simulink subsystem "EnergyElectroThermal"  (R2023b)
settings: Solver=VariableStepAuto  StartTime=0.0  StopTime=10.0  RelTol=1e-3
settings Model: Creator=jjha  LastModifiedBy=jjha

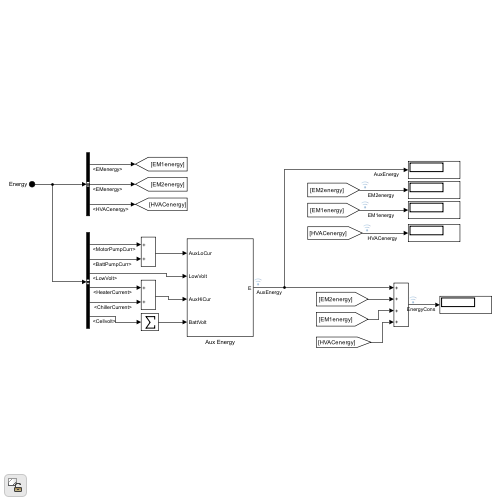
[thumbnail: Simulink's stored preview of the top-level diagram]
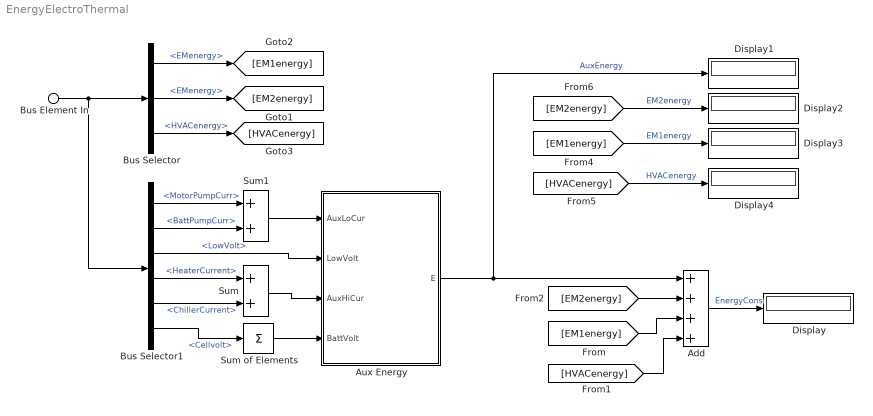
== system EnergyElectroThermal ==
  Bus Element In : Inport  PortName=Energy
  Add : Sum  Inputs=++++
  Aux Energy : Subsystem
  Bus Selector : BusSelector  OutputSignals=M1.EMenergy,M2.EMenergy,VA.HVACenergy
  Bus Selector1 : BusSelector  OutputSignals=MP.MotorPumpCurr,BP.BattPumpCurr,MP.LowVolt,HE.HeaterCurrent,CH.ChillerCurrent,BA.BattSens.Cellvolt
  Display{,1..4} (5 alike) : Display
  Sum : Sum
  Sum of Elements : Sum  Inputs=+
  Sum1 : Sum
  wires:
  [EM2energy] -> Add/2
  [EM1energy] -> Add/3
  [HVACenergy] -> Add/4
  Add/1 -> Display/1  "EnergyCons"
  Aux Energy/1(E) -> Add/1, Display1/1  "AuxEnergy"
  [EM2energy] -> Display2/1  "EM2energy"
  [EM1energy] -> Display3/1  "EM1energy"
  [HVACenergy] -> Display4/1  "HVACenergy"
  Bus Selector/3 -> [HVACenergy]  "<HVACenergy>"
  Bus Element In/1 -> Bus Selector1/1, Bus Selector/1
  Bus Selector1/5 -> Sum/2  "<ChillerCurrent>"
  Bus Selector1/3 -> Aux Energy/2(LowVolt)  "<LowVolt>"
  Sum1/1 -> Aux Energy/1(AuxLoCur)
  Sum/1 -> Aux Energy/3(AuxHiCur)
  Bus Selector1/4 -> Sum/1  "<HeaterCurrent>"
  Bus Selector1/1 -> Sum1/1  "<MotorPumpCurr>"
  Bus Selector1/2 -> Sum1/2  "<BattPumpCurr>"
  Bus Selector1/6 -> Sum of Elements/1  "<Cellvolt>"
  Sum of Elements/1 -> Aux Energy/4(BattVolt)
  Bus Selector/2 -> [EM2energy]  "<EMenergy>"
  Bus Selector/1 -> [EM1energy]  "<EMenergy>"

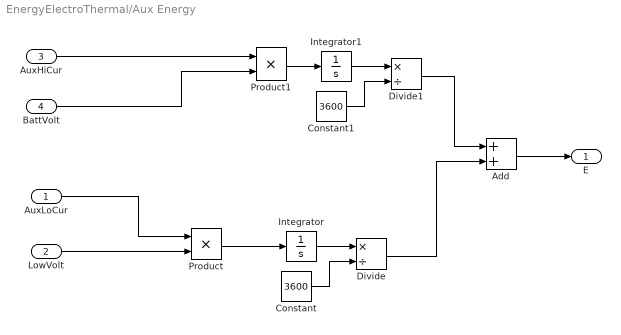
== system EnergyElectroThermal/Aux Energy ==
  AuxLoCur : Inport
  LowVolt : Inport  Port=2
  AuxHiCur : Inport  Port=3
  BattVolt : Inport  Port=4
  Add : Sum
  Constant : Constant  Value=3600
  Constant1 : Constant  Value=3600
  Divide : Product  Inputs=*/
  Divide1 : Product  Inputs=*/
  Integrator : Integrator  ZeroCross=off
  Integrator1 : Integrator  ZeroCross=off
  Product : Product
  Product1 : Product
  E : Outport
  wires:
  BattVolt/1 -> Product1/2
  Divide/1 -> Add/2
  Divide1/1 -> Add/1
  Product1/1 -> Integrator1/1
  Constant1/1 -> Divide1/2
  Integrator1/1 -> Divide1/1
  AuxHiCur/1 -> Product1/1
  Product/1 -> Integrator/1
  Integrator/1 -> Divide/1
  Constant/1 -> Divide/2
  LowVolt/1 -> Product/2
  Add/1 -> E/1
  AuxLoCur/1 -> Product/1
